simulink model "p4_car_Luke_ind1"  (R2025a)
settings: Solver=ode5  StartTime=0.0  StopTime=3600  FixedStep=0.005  RelTol=1e-3
undefined symbols (not defined in the file or in its folder): datBat, datCar, datMotor, path
libraries: slpidlib x1
(part 2 of 2)

== matlab function p4_car_Luke_ind1/Environment/MATLAB Function ==
  data: x input; grade output; y input
function grade = fcn(x, y)
slope = 0;
if x>=0 && x<=900 && y<20 %bottom straightway
    h = exp((x-450)/50) / (1 + exp((x-450)/50)) * 10;
    slope = (10/50) * exp((x-450)/50) ./ (1 + exp((x-450)/50)).^2;
elseif x>=0 && x<=900 && y>20 %top straightaway
    h = exp((450-x)/50) / (1 + exp((450-x)/50)) * 10;
    slope = -exp((450-x)/50) ./ (5 * (1 + exp((450-x)/50)).^2);

elseif x>900 %right curve
    h=10; %max height from funciton
    slope = 0
elseif x<0 %left curve
    h=0; %min height
    slope = 0;
end

grade = slope;

== matlab function p4_car_Luke_ind1/Race Car/Longitudinal Dynamics Body Frame/Electric Motor Drive/Electric Motor/MATLAB Function1 ==
  data: Tm input; I_bus output; Wm input; Effm input; V_bus input
function I_bus = fcn(Tm, Wm, Effm, V_bus)
    Pm = Tm*Wm;
    sgn_m = Pm / (abs(Pm) + 0.001);
    Pe = Pm / (Effm^sgn_m);
    if V_bus > 1
        I_bus = Pe/V_bus;
    else
        I_bus = 0;
    end

== matlab function p4_car_Luke_ind1/Race Car/Longitudinal Dynamics Body Frame/Wheel /MATLAB Function ==
  data: r_w input; v_w input; omega_w input; lambda output
function lambda = tire_slip_ratio(r_w, v_w, omega_w)
% r_w - wheel radius
% v_w - wheel axle speed (m/s)
% omega_w - wheel speed (rad/s)
% lambda - tire slip ratio

epsilon = 0.0001; % a small number for numerical smoothening

if (r_w * omega_w >= v_w - epsilon)
    lambda = (r_w * omega_w - v_w) / (abs(r_w * omega_w) + epsilon);
else
    lambda = (r_w * omega_w - v_w) / (abs(v_w) + epsilon);
end

== matlab function p4_car_Luke_ind1/Race Car/Longitudinal Dynamics Body Frame/Wheel /MATLAB Function1 ==
  data: tau_axle input; alpha_w output; tau_brake input; I_in input; I_w input; r_w input; F_x input
function alpha_w = wheel_acceleration(tau_axle, tau_brake, I_in, I_w, r_w, F_x)
% tau_axle - axle torque (Nm)
% tau_brake - brake torque (Nm)
% I_in - input inertia (Kg m^2)
% I_w - wheel inertia (Kg m^2)
% r_w - tire radius (m)
% F_x - tractive force from tire contact (N)
% alpha_w = wheel (angular) acceleration (rad / s^2)

alpha_w = (tau_axle - tau_brake - F_x * r_w ) / (I_in + I_w);

== matlab function p4_car_Luke_ind1/Race Car/Longitudinal Dynamics Body Frame/Wheel /MATLAB Function2 ==
  data: lambda input; F_x output; lambda_max input; nominal_stiffness input; mu input; mass input
function F_x = tire_tractive_force(lambda, lambda_max, nominal_stiffness, mu, mass )
% lambda - tire slip ratio
% lambda_max - maximum tire slip ratio for F_x calculations
% nominal_stiffness - tire long stiffness (N)
% mu - (effective) friction coefficient - in the range [0, 1]
% mass - vehicle mass for normal force calculation

g = 9.81; % gravity - m/ s^2

N = mass * g/4;  % assume 4 tires and equal distribution across tires

C_lambda = nominal_stiffness * mu * N;
if lambda >= 0
    F_x = C_lambda * min(lambda_max, lambda);
else
    F_x = C_lambda * max(-lambda_max, lambda);
end

== matlab function p4_car_Luke_ind1/Race Car/Longitudinal Dynamics Body Frame/Electric Motor Drive/Inverter/Inverter Calculations ==
  data: V_bat input; Eff_I input; V_bus output; I_bus input; I_bat output
function [V_bus, I_bat] = fcn(V_bat, Eff_I, I_bus)
    V_bus = V_bat; % Vbus = Vbat * r, where r is the inverter conversion ratio % * I_bat * Eff_I^(sgn_Pbat))/ I_bus;
    P_bus = V_bus *I_bus;
    sgn_Pbus = P_bus / (abs(P_bus) + 0.001);
    
    if V_bat > 1
        I_bat = (P_bus / Eff_I^sgn_Pbus) / V_bat ;
    else
        I_bat = 0;
    end

end

% double check

== matlab function p4_car_Luke_ind1/Race Car/CarKinematicsInertialFrame/KinematicVehicleModel_derivatives ==
  data: vx input; vy input; psi input size=1; Xdot output; Ydot output
function [Xdot, Ydot] = fcn(vx, vy, psi)
    temp = TF(psi) * [vx;vy]; 
    Xdot = temp(1);
    Ydot = temp(2);
  
end

function y = TF(psi)
    y = [cos(psi), -sin(psi); sin(psi), cos(psi)];
end

== matlab function p4_car_Luke_ind1/Race Car/Longitudinal Dynamics Body Frame/Brake System/Brake Torque ==
  data: BBcmd input; Tbcap input; Tb output; w_wheel input
function Tb = fcn(BBcmd, Tbcap, w_wheel)
% DESCRIPTION: 
%   This function takes the brake torque capacity, the angular velocity of
%   the wheel. A simple approximation for the brake torque capacity is 
%   the brake command times some calibratable constant 

% INPUTS:
%   BBcmd - brake percent command
%   Tbcap - brake torque capacity  [N-m]
%   w_wheel - wheels angular velocity [rad/s]

% OUTPUTS:
%   Tb - actual brake torque [N-m]

Tb = -BBcmd * Tbcap * (w_wheel / (abs(w_wheel) + 0.001));

end
